simulink model "et_robocon_dev_guy"  (R2013b)
settings: Solver=FixedStepDiscrete  SolverMode=SingleTasking  StartTime=0.0  StopTime=inf  FixedStep=balancer_ts  RelTol=1e-3
undefined symbols (not defined in the file): a_d, a_r, balancerStates_Bus0, Batt, battery_gain, battery_offset, cmd_max, current_mode_status, current_task_operation_status, DiscIntNeverNeededParam, exec_period, Init_Bus0, k_f, k_i, k_phidot, k_thetadot, lightCalib, R, STATE, TRACK_MODE_LIST, ts2, W
libraries: simulink x29, legonxtlib x28, simulink_extras x4, light_sensor_calibration_algorithm_atomic_sub_chart_library x3, gyro_calibration_algorithm_atomic_sub_chart_library x1, limbo_algorithm_atomic_sub_chart_library x1, see_saw x1
(part 3 of 3)

== system et_robocon_dev_guy/Main Controller/normal_operation_modes.line_tracking_mode/line_tracking_mode.processLight/LineTracePID/SwitchController/BasicStage/6thCorner/SpeedUp ==
  TargetFwd : Inport
  LastFwd : Inport  Port=2
  Constant1 : Constant  Value=2  OutDataTypeStr=single  SampleTime=-1
  Saturation1 : Saturate  UpperLimit=160  LowerLimit=80  RndMeth=Simplest
  Sum1 : Sum  Inputs=-+  AccumDataTypeStr=single  OutDataTypeStr=single  RndMeth=Simplest
  Sum2 : Sum  Inputs=|++  AccumDataTypeStr=single  OutDataTypeStr=single  RndMeth=Simplest  InputSameDT=on
  Sum3 : Sum  Inputs=|++  AccumDataTypeStr=single  OutDataTypeStr=single  RndMeth=Simplest  InputSameDT=on
  Switch : Switch  Criteria=u2 > Threshold  OutDataTypeStr=single  RndMeth=Simplest
  Unit Delay1 : UnitDelay  SampleTime=-1
  fwd : Outport
  wires:
  TargetFwd/1 -> Switch/1, Sum1/1
  Switch/1 -> fwd/1
  Sum1/1 -> Switch/2
  Unit Delay1/1 -> Sum2/2
  LastFwd/1 -> Sum3/1
  Constant1/1 -> Sum2/1
  Sum3/1 -> Saturation1/1
  Saturation1/1 -> Switch/3, Sum1/2
  Sum2/1 -> Sum3/2, Unit Delay1/1

== system et_robocon_dev_guy/Main Controller/normal_operation_modes.line_tracking_mode/line_tracking_mode.processLight/LineTracePID/SwitchController/BasicStage/CenterStraight/Normal ==
  note: Max_chargingFwd
  note: speed up (or) speed down counter
  Fwd : Inport
  Constant2 : Constant  Value=0  OutDataTypeStr=single  SampleTime=-1
  Constant4 : Constant  Value=140  OutDataTypeStr=single  SampleTime=-1
  MinMax : MinMax  Function=max
  MinMax1 : MinMax
  Mux : Mux  Inputs=2
  Product : Product  Inputs=*/
  Saturation : Saturate  UpperLimit=10  LowerLimit=-10
  Saturation Dynamic : simulink/Discontinuities/Saturation Dynamic  OutMin=[]  OutMax=[]  OutDataTypeStr=Inherit: Same as second input  OutDataType=fixdt(1, 16)  OutScaling=2^-10  DoSatur=off
  Signal Conversion : SignalConversion
  Sum4 : Sum  Inputs=|+-  AccumDataTypeStr=single  OutDataTypeStr=single  RndMeth=Simplest  InputSameDT=on
  Sum5 : Sum  Inputs=|++  AccumDataTypeStr=single  OutDataTypeStr=single  RndMeth=Simplest  InputSameDT=on
  Unit Delay External IC : simulink/Additional Math & Discrete/Additional Discrete/Unit Delay External IC  tsamp=-1
  steps for rising/falling : Constant  Value=70  OutDataTypeStr=single
  Out1 : Outport
  fwd : Outport  Port=2
  wires:
  Constant2/1 -> Out1/1
  Fwd/1 -> Unit Delay External IC/2, Sum4/2, Mux/2
  Sum4/1 -> Product/1
  Constant4/1 -> Sum4/1, Mux/1
  Sum5/1 -> Saturation Dynamic/2, Unit Delay External IC/1
  Unit Delay External IC/1 -> Sum5/1
  Product/1 -> Saturation/1
  steps for rising/falling/1 -> Product/2
  Mux/1 -> MinMax1/1, MinMax/1
  MinMax/1 -> Saturation Dynamic/1
  MinMax1/1 -> Saturation Dynamic/3
  Saturation/1 -> Sum5/2
  Saturation Dynamic/1 -> Signal Conversion/1
  Signal Conversion/1 -> fwd/1

== system et_robocon_dev_guy/Main Controller/normal_operation_modes.line_tracking_mode/line_tracking_mode.processLight/LineTracePID/SwitchController/BasicStage/CenterStraight/Speak ==
  Enable : EnablePort
  Constant : Constant  Value=50
  Speaker : legonxtlib/Speaker  sinputMode=Volume only  sspeakerFreq=800  sspeakerVolume=50  sspeakerDuration=100
  wires:
  Constant/1 -> Speaker/1

== system et_robocon_dev_guy/Main Controller/normal_operation_modes.line_tracking_mode/line_tracking_mode.processLight/LineTracePID/SwitchController/BasicStage/LastStraight/Normal ==
  note: Max_chargingFwd
  note: speed up (or) speed down counter
  Fwd : Inport
  Constant2 : Constant  Value=0  OutDataTypeStr=single  SampleTime=-1
  Constant4 : Constant  Value=140  OutDataTypeStr=single  SampleTime=-1
  MinMax : MinMax  Function=max
  MinMax1 : MinMax
  Mux : Mux  Inputs=2
  Product : Product  Inputs=*/
  Saturation : Saturate  UpperLimit=10  LowerLimit=-10
  Saturation Dynamic : simulink/Discontinuities/Saturation Dynamic  OutMin=[]  OutMax=[]  OutDataTypeStr=Inherit: Same as second input  OutDataType=fixdt(1, 16)  OutScaling=2^-10  DoSatur=off
  Signal Conversion : SignalConversion
  Sum4 : Sum  Inputs=|+-  AccumDataTypeStr=single  OutDataTypeStr=single  RndMeth=Simplest  InputSameDT=on
  Sum5 : Sum  Inputs=|++  AccumDataTypeStr=single  OutDataTypeStr=single  RndMeth=Simplest  InputSameDT=on
  Unit Delay External IC : simulink/Additional Math & Discrete/Additional Discrete/Unit Delay External IC  tsamp=-1
  steps for rising/falling : Constant  Value=60  OutDataTypeStr=single
  Out1 : Outport
  fwd : Outport  Port=2
  wires:
  Constant2/1 -> Out1/1
  Fwd/1 -> Unit Delay External IC/2, Sum4/2, Mux/2
  Sum4/1 -> Product/1
  Constant4/1 -> Sum4/1, Mux/1
  Sum5/1 -> Saturation Dynamic/2, Unit Delay External IC/1
  Unit Delay External IC/1 -> Sum5/1
  Product/1 -> Saturation/1
  steps for rising/falling/1 -> Product/2
  Mux/1 -> MinMax1/1, MinMax/1
  MinMax/1 -> Saturation Dynamic/1
  MinMax1/1 -> Saturation Dynamic/3
  Saturation/1 -> Sum5/2
  Saturation Dynamic/1 -> Signal Conversion/1
  Signal Conversion/1 -> fwd/1

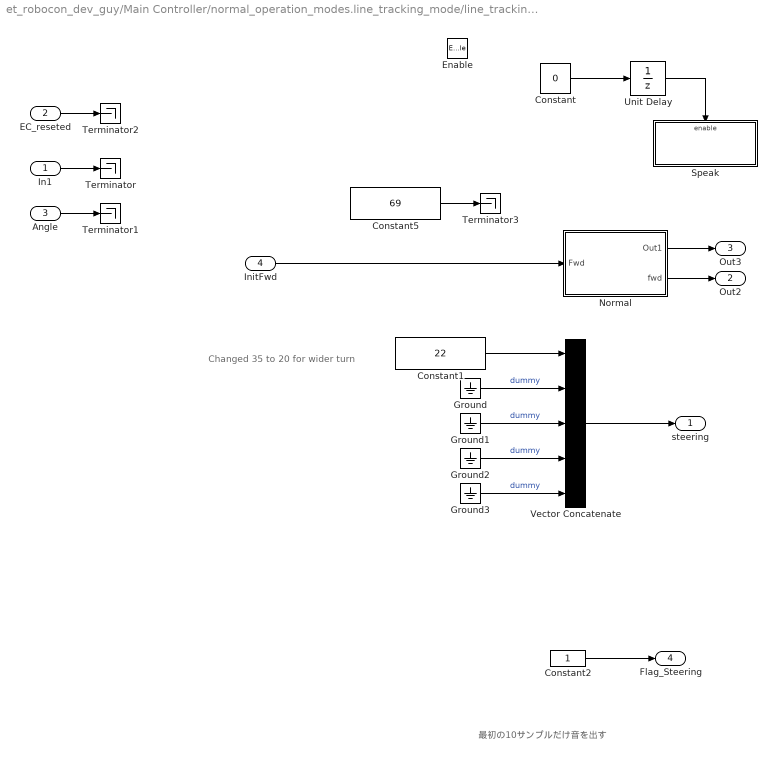
== system et_robocon_dev_guy/Main Controller/normal_operation_modes.line_tracking_mode/line_tracking_mode.processLight/LineTracePID/SwitchController/BasicStage/ShortCut/BlindRun ==
  note: Changed 35 to 20 for wider turn
  note: 最初の10サンプルだけ音を出す
  In1 : Inport
  EC_reseted : Inport  Port=2
  Angle : Inport  Port=3
  InitFwd : Inport  Port=4
  Enable : EnablePort
  Constant : Constant  Value=0
  Constant1 : Constant  Value=22  OutDataTypeStr=single  SampleTime=-1
  Constant2 : Constant  OutDataTypeStr=single  SampleTime=-1
  Constant5 : Constant  Value=69  OutDataTypeStr=single  SampleTime=-1
  Ground{,1..3} (4 alike) : Ground
  Normal : Subsystem  TreatAsAtomicUnit=on
  Speak : Subsystem  TreatAsAtomicUnit=on
  Terminator{,1..3} (4 alike) : Terminator
  Unit Delay : UnitDelay  InitialCondition=1  SampleTime=-1
  Vector Concatenate : Concatenate  NumInputs=5
  steering : Outport
  Out2 : Outport  Port=2
  Out3 : Outport  Port=3
  Flag_Steering : Outport  Port=4
  wires:
  In1/1 -> Terminator/1
  Angle/1 -> Terminator1/1
  EC_reseted/1 -> Terminator2/1
  Normal/2(fwd) -> Out2/1
  Normal/1(Out1) -> Out3/1
  Vector Concatenate/1 -> steering/1
  Ground/1 -> Vector Concatenate/2  "dummy"
  Ground1/1 -> Vector Concatenate/3  "dummy"
  Ground2/1 -> Vector Concatenate/4  "dummy"
  Ground3/1 -> Vector Concatenate/5  "dummy"
  Constant2/1 -> Flag_Steering/1
  Constant5/1 -> Terminator3/1
  InitFwd/1 -> Normal/1(Fwd)
  Constant1/1 -> Vector Concatenate/1
  Constant/1 -> Unit Delay/1
  Unit Delay/1 -> Speak/Enable

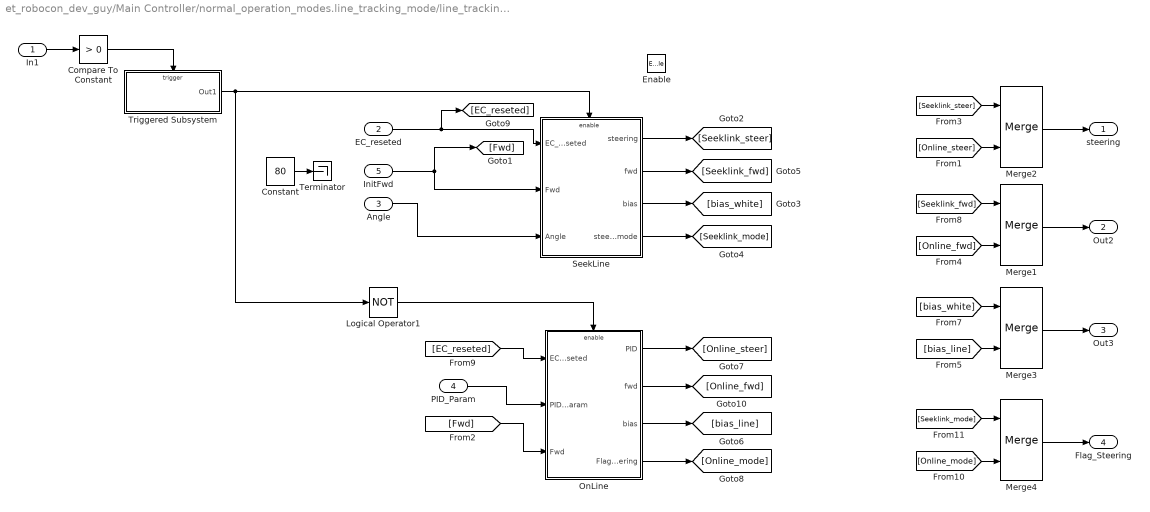
== system et_robocon_dev_guy/Main Controller/normal_operation_modes.line_tracking_mode/line_tracking_mode.processLight/LineTracePID/SwitchController/BasicStage/ShortCut/SeekAndPIDRun ==
  In1 : Inport
  EC_reseted : Inport  Port=2
  Angle : Inport  Port=3
  PID_Param : Inport  Port=4
  InitFwd : Inport  Port=5
  Enable : EnablePort
  Compare To Constant : simulink/Logic and Bit Operations/Compare To Constant  relop=>  const=0  OutDataTypeStr=boolean
  Constant : Constant  Value=80  OutDataTypeStr=single
  Logical Operator1 : Logic  Operator=NOT  AllPortsSameDT=off  OutDataTypeStr=boolean
  Merge{1..4} (4 alike) : Merge
  OnLine : Subsystem  TreatAsAtomicUnit=on
  SeekLine : Subsystem  TreatAsAtomicUnit=on
  Terminator : Terminator
  Triggered Subsystem : Subsystem  TreatAsAtomicUnit=on
  steering : Outport
  Out2 : Outport  Port=2
  Out3 : Outport  Port=3
  Flag_Steering : Outport  Port=4
  wires:
  [bias_line] -> Merge3/2
  [bias_white] -> Merge3/1
  OnLine/3(bias) -> [bias_line]
  SeekLine/3(bias) -> [bias_white]
  PID_Param/1 -> OnLine/2(PID_Param)
  [EC_reseted] -> OnLine/1(EC_reseted)
  Logical Operator1/1 -> OnLine/Enable
  Angle/1 -> SeekLine/3(Angle)
  EC_reseted/1 -> SeekLine/1(EC_reseted), [EC_reseted]
  Merge1/1 -> Out2/1
  Merge3/1 -> Out3/1
  Merge2/1 -> steering/1
  Merge4/1 -> Flag_Steering/1
  Compare To Constant/1 -> Triggered Subsystem/Trigger
  Triggered Subsystem/1(Out1) -> SeekLine/Enable, Logical Operator1/1
  [Fwd] -> OnLine/3(Fwd)
  In1/1 -> Compare To Constant/1
  SeekLine/1(steering) -> [Seeklink_steer]
  SeekLine/2(fwd) -> [Seeklink_fwd]
  SeekLine/4(steering_mode) -> [Seeklink_mode]
  [Seeklink_steer] -> Merge2/1
  [Online_steer] -> Merge2/2
  [Seeklink_fwd] -> Merge1/1
  [Online_fwd] -> Merge1/2
  [Seeklink_mode] -> Merge4/1
  [Online_mode] -> Merge4/2
  OnLine/1(PID) -> [Online_steer]
  OnLine/2(fwd) -> [Online_fwd]
  OnLine/4(Flag_Steering) -> [Online_mode]
  InitFwd/1 -> [Fwd], SeekLine/2(Fwd)
  Constant/1 -> Terminator/1

== system et_robocon_dev_guy/Main Controller/normal_operation_modes.line_tracking_mode/line_tracking_mode.processLight/LineTracePID/SwitchController/BasicStage/ShortCut/Triggered Subsystem ==
  Trigger : TriggerPort
  Constant : Constant  Value=0  OutDataTypeStr=boolean
  Out1 : Outport  InitialOutput=[1]
  wires:
  Constant/1 -> Out1/1

== system et_robocon_dev_guy/Main Controller/normal_operation_modes.line_tracking_mode/line_tracking_mode.processLight/LineTracePID/SwitchController/BasicStage/Slope/Slope Mode 0 ==
  Fwd : Inport
  Bias : Inport  Port=2
  Action Port : ActionPort  ActionType=default
  bias : Outport
  fwd : Outport  Port=2
  wires:
  Bias/1 -> bias/1
  Fwd/1 -> fwd/1

== system et_robocon_dev_guy/Main Controller/normal_operation_modes.line_tracking_mode/line_tracking_mode.processLight/LineTracePID/SwitchController/BasicStage/Slope/Slope Mode 1 ==
  Fwd : Inport
  Bias : Inport  Port=2
  PreFwd : Inport  Port=3
  Action Port : ActionPort  ActionType=case
  Constant : Constant  Value=-1  OutDataTypeStr=single
  Saturation Dynamic : simulink/Discontinuities/Saturation Dynamic  OutMin=[]  OutMax=[]  OutDataTypeStr=Inherit: Same as second input  OutDataType=fixdt(1, 16)  OutScaling=2^-10  DoSatur=off
  Signal Conversion : SignalConversion
  Sum : Sum  Inputs=|++
  Sum1 : Sum  Inputs=|++
  Unit Delay : UnitDelay  SampleTime=-1
  bias : Outport
  fwd : Outport  Port=2
  wires:
  Bias/1 -> bias/1
  Fwd/1 -> Saturation Dynamic/3
  Constant/1 -> Sum/1
  Sum/1 -> Unit Delay/1, Sum1/2
  Sum1/1 -> Saturation Dynamic/2
  Saturation Dynamic/1 -> Signal Conversion/1
  PreFwd/1 -> Saturation Dynamic/1, Sum1/1
  Signal Conversion/1 -> fwd/1
  Unit Delay/1 -> Sum/2

== system et_robocon_dev_guy/Main Controller/normal_operation_modes.line_tracking_mode/line_tracking_mode.processLight/LineTracePID/SwitchController/BasicStage/Slope/Slope Mode 2 ==
  Fwd : Inport
  Bias : Inport  Port=2
  PreFwd : Inport  Port=3
  Action Port : ActionPort  ActionType=case
  Constant : Constant  OutDataTypeStr=single
  Saturation Dynamic : simulink/Discontinuities/Saturation Dynamic  OutMin=[]  OutMax=[]  OutDataTypeStr=Inherit: Same as second input  OutDataType=fixdt(1, 16)  OutScaling=2^-10  DoSatur=off
  Signal Conversion : SignalConversion
  Sum : Sum  Inputs=|++
  Sum1 : Sum  Inputs=|++
  Unit Delay : UnitDelay  SampleTime=-1
  bias : Outport
  fwd : Outport  Port=2
  wires:
  Bias/1 -> bias/1
  Constant/1 -> Sum/1
  Sum/1 -> Unit Delay/1, Sum1/2
  Sum1/1 -> Saturation Dynamic/2
  Saturation Dynamic/1 -> Signal Conversion/1
  PreFwd/1 -> Saturation Dynamic/1, Sum1/1
  Fwd/1 -> Saturation Dynamic/3
  Signal Conversion/1 -> fwd/1
  Unit Delay/1 -> Sum/2

== system et_robocon_dev_guy/Main Controller/normal_operation_modes.line_tracking_mode/line_tracking_mode.processLight/LineTracePID/SwitchController/BonusStage/Gate/Normal ==
  Fwd : Inport
  Constant2 : Constant  Value=-10  OutDataTypeStr=single  SampleTime=-1
  Out1 : Outport
  fwd : Outport  Port=2
  wires:
  Fwd/1 -> fwd/1
  Constant2/1 -> Out1/1

== system et_robocon_dev_guy/Main Controller/normal_operation_modes.line_tracking_mode/line_tracking_mode.processLight/LineTracePID/SwitchController/BonusStage/Gate/SlowDown ==
  TargetFwd : Inport
  LastFwd : Inport  Port=2
  Constant1 : Constant  Value=-0.5  OutDataTypeStr=single  SampleTime=-1
  Saturation1 : Saturate  UpperLimit=160  LowerLimit=0  RndMeth=Simplest
  Sum1 : Sum  Inputs=+-  AccumDataTypeStr=single  OutDataTypeStr=single  RndMeth=Simplest
  Sum2 : Sum  Inputs=|++  AccumDataTypeStr=single  OutDataTypeStr=single  RndMeth=Simplest  InputSameDT=on
  Sum3 : Sum  Inputs=|++  AccumDataTypeStr=single  OutDataTypeStr=single  RndMeth=Simplest  InputSameDT=on
  Switch : Switch  Criteria=u2 > Threshold  OutDataTypeStr=single  RndMeth=Simplest
  Unit Delay1 : UnitDelay  SampleTime=-1
  fwd : Outport
  wires:
  TargetFwd/1 -> Switch/1, Sum1/1
  Switch/1 -> fwd/1
  Sum1/1 -> Switch/2
  Unit Delay1/1 -> Sum2/2
  LastFwd/1 -> Sum3/1
  Constant1/1 -> Sum2/1
  Sum3/1 -> Saturation1/1
  Saturation1/1 -> Switch/3, Sum1/2
  Sum2/1 -> Sum3/2, Unit Delay1/1

== system et_robocon_dev_guy/Main Controller/normal_operation_modes.line_tracking_mode/line_tracking_mode.processLight/LineTracePID/SwitchController/BonusStage/IntoGarage/Normal ==
  Fwd : Inport
  Constant2 : Constant  Value=-10  OutDataTypeStr=single  SampleTime=-1
  Out1 : Outport
  fwd : Outport  Port=2
  wires:
  Constant2/1 -> Out1/1
  Fwd/1 -> fwd/1

== system et_robocon_dev_guy/Main Controller/normal_operation_modes.line_tracking_mode/line_tracking_mode.processLight/LineTracePID/SwitchController/BasicStage/ShortCut/BlindRun/Normal ==
  Fwd : Inport
  Constant2 : Constant  Value=0  OutDataTypeStr=single  SampleTime=-1
  Out1 : Outport
  fwd : Outport  Port=2
  wires:
  Constant2/1 -> Out1/1
  Fwd/1 -> fwd/1

== system et_robocon_dev_guy/Main Controller/normal_operation_modes.line_tracking_mode/line_tracking_mode.processLight/LineTracePID/SwitchController/BasicStage/ShortCut/BlindRun/Speak ==
  Enable : EnablePort
  Constant : Constant  Value=50
  Speaker : legonxtlib/Speaker  sinputMode=Volume only  sspeakerFreq=800  sspeakerVolume=50  sspeakerDuration=100
  wires:
  Constant/1 -> Speaker/1

== system et_robocon_dev_guy/Main Controller/normal_operation_modes.line_tracking_mode/line_tracking_mode.processLight/LineTracePID/SwitchController/BasicStage/ShortCut/SeekAndPIDRun/OnLine ==
  note: 最初の10サンプルだけ音を出す
  EC_reseted : Inport
  PID_Param : Inport  Port=2
  Fwd : Inport  Port=3
  Enable : EnablePort
  Constant : Constant  Value=0.2  OutDataTypeStr=single
  Constant1 : Constant  Value=0  OutDataTypeStr=single  SampleTime=-1
  Constant2 : Constant  Value=5  OutDataTypeStr=single  SampleTime=-1
  Constant3 : Constant  Value=0
  Saturation : Saturate  UpperLimit=140  LowerLimit=0
  Speak : Subsystem  TreatAsAtomicUnit=on
  Sum : Sum  Inputs=|++
  Sum1 : Sum  Inputs=|++
  Terminator : Terminator
  Unit Delay : UnitDelay  SampleTime=-1
  Unit Delay1 : UnitDelay  InitialCondition=1  SampleTime=-1
  PID : Outport
  fwd : Outport  Port=2
  bias : Outport  Port=3
  Flag_Steering : Outport  Port=4
  wires:
  Constant2/1 -> bias/1
  PID_Param/1 -> PID/1
  EC_reseted/1 -> Terminator/1
  Fwd/1 -> Sum1/1
  Sum1/1 -> Saturation/1
  Sum/1 -> Unit Delay/1, Sum1/2
  Unit Delay/1 -> Sum/2
  Saturation/1 -> fwd/1
  Constant1/1 -> Flag_Steering/1
  Constant/1 -> Sum/1
  Constant3/1 -> Unit Delay1/1
  Unit Delay1/1 -> Speak/Enable

== system et_robocon_dev_guy/Main Controller/normal_operation_modes.line_tracking_mode/line_tracking_mode.processLight/LineTracePID/SwitchController/BasicStage/ShortCut/SeekAndPIDRun/SeekLine ==
  note: Change -7 to -3
  EC_reseted : Inport
  Fwd : Inport  Port=2
  Angle : Inport  Port=3
  Enable : EnablePort
  Constant : Constant  Value=-3  OutDataTypeStr=single
  Constant1 : Constant  OutDataTypeStr=single  SampleTime=-1
  Constant2 : Constant  Value=0  OutDataTypeStr=single  SampleTime=-1
  Constant3 : Constant  Value=-10  OutDataTypeStr=single
  Constant4 : Constant  Value=0
  Ground{,1..3} (4 alike) : Ground
  Speak : Subsystem  TreatAsAtomicUnit=on
  Terminator : Terminator
  Terminator1 : Terminator
  Terminator2 : Terminator
  Unit Delay : UnitDelay  InitialCondition=1  SampleTime=-1
  Vector Concatenate : Concatenate  NumInputs=5
  steering : Outport
  fwd : Outport  Port=2
  bias : Outport  Port=3
  steering_mode : Outport  Port=4
  wires:
  Angle/1 -> Terminator1/1
  EC_reseted/1 -> Terminator/1
  Fwd/1 -> fwd/1
  Constant2/1 -> bias/1
  Ground/1 -> Vector Concatenate/2  "dummy"
  Ground1/1 -> Vector Concatenate/3  "dummy"
  Ground2/1 -> Vector Concatenate/4  "dummy"
  Ground3/1 -> Vector Concatenate/5  "dummy"
  Vector Concatenate/1 -> steering/1
  Constant1/1 -> steering_mode/1
  Constant/1 -> Vector Concatenate/1
  Constant3/1 -> Terminator2/1
  Constant4/1 -> Unit Delay/1
  Unit Delay/1 -> Speak/Enable

== system et_robocon_dev_guy/Main Controller/normal_operation_modes.line_tracking_mode/line_tracking_mode.processLight/LineTracePID/SwitchController/BasicStage/ShortCut/SeekAndPIDRun/Triggered Subsystem ==
  Trigger : TriggerPort
  Constant : Constant  Value=0  OutDataTypeStr=boolean
  Out1 : Outport  InitialOutput=[1]
  wires:
  Constant/1 -> Out1/1

== system et_robocon_dev_guy/Main Controller/normal_operation_modes.line_tracking_mode/line_tracking_mode.processLight/LineTracePID/SwitchController/BasicStage/ShortCut/SeekAndPIDRun/OnLine/Speak ==
  Enable : EnablePort
  Constant : Constant  Value=50
  Speaker : legonxtlib/Speaker  sinputMode=Volume only  sspeakerFreq=800  sspeakerVolume=50  sspeakerDuration=100
  wires:
  Constant/1 -> Speaker/1

== system et_robocon_dev_guy/Main Controller/normal_operation_modes.line_tracking_mode/line_tracking_mode.processLight/LineTracePID/SwitchController/BasicStage/ShortCut/SeekAndPIDRun/SeekLine/Speak ==
  Enable : EnablePort
  Constant : Constant  Value=50
  Speaker : legonxtlib/Speaker  sinputMode=Volume only  sspeakerFreq=800  sspeakerVolume=50  sspeakerDuration=100
  wires:
  Constant/1 -> Speaker/1

== stateflow chart et_robocon_dev_guy/State Estimation/Gyro Processing/Reset Subsystem ==
  state CheckForReset
    bind: doProcess;
    entry: doProcess;
    during: doProcess;
  (default) -> CheckForReset
  CheckForReset -> CheckForReset : [init_flag == 1]
  data: init_flag input
  events: doProcess output FUNCTION_CALL_EVENT

== stateflow chart et_robocon_dev_guy/Main Controller/normal_operation_modes.line_tracking_mode ==
  state line_tracking_mode
    entry:
    desired_tail = single(0); %radian
    entry, during:
    PWM.tail = tail_controller(sensors.theta_T,desired_tail);
    exit:
    PWM.tail = single(0);
    state Waiting
      entry: debugFlag = uint16(400);
    state Track
      entry:
      debugFlag = uint16(401);
      during:
      on every(3, tick):  lineTrackCmd = processLight(rawSensors);
      during:
      [PWM.left PWM.right] = balanceControl(rawSensors,lineTrackCmd);
    state Stop
      entry:
      speed_ref = lineTrackCmd(1);
      during:
      lineTrackCmd = single([speed_ref 0]');
      [PWM.left PWM.right] = balanceControl(rawSensors,lineTrackCmd);
      desired_tail = single(1.6); %radian
      speed_ref = speed_ref - single(1);
    state Kick
      entry:
      PWM.left = single(100)
      PWM.right = single(100);
      exit:
      PWM.left = single(0)
      PWM.right = single(0);
    state Done
      entry:
      turnLightOn;
      debugFlag = uint16(402);
      PWM.left = single(0); PWM.right = single(0);
      current_mode_status = OperationModeStatusEnum.SUCCESSFULLY_COMPLETED;
    state turnLightOn [function]
    state lineTrackCmd = processLight(rawSensors) [function]
    state [leftPWM,rightPWM]  = balanceControl(rawSensors, lineTrackCmd) [function]
    state cmd = tail_controller(current,desired) [function]
    (default) -> Waiting
    Waiting -> Track : [hasChangedFrom(touch,single(0))]
    Track -> Stop : [(sensors.theta_L + sensors.theta_R)/2>single(320)]
    Stop -> Kick : [speed_ref<0]
    Kick -> Done : after(0.2,sec)
  data: lineTrackCmd function_output single size=2; rawSensors function_input Bus: Sensors_Bus size=1; leftPWM function_output single size=1; rawSensors function_input Bus: Sensors_Bus size=1; rightPWM function_output; lineTrackCmd function_input single size=2; current function_input single size=1; desired function_input single size=1; cmd function_output single size=1; sensors input Bus: Sensors_Bus size=1; lightCalib data_store_memory size=1; touch input single size=1; PWM output Bus: PWM_bus size=1; debugFlag output uint16 size=1; current_mode_status data_store_memory; desired_tail local single size=1; speed_ref local single size=1; states input Bus: States_Bus size=1; rawSensors input Bus: Sensors_Bus size=1; lineTrackCmd local single size=2

== stateflow chart et_robocon_dev_guy/State Estimation/StateEstimation/Reset Subsystem ==
  state CheckForReset
    bind: doProcess;
    entry: doProcess;
    during: doProcess;
  (default) -> CheckForReset
  CheckForReset -> CheckForReset : [init_flag == 1]
  data: init_flag input
  events: doProcess output FUNCTION_CALL_EVENT

== stateflow chart et_robocon_dev_guy/Main Controller ==
  state restore
  state emergency_stop
    entry:
    debugFlag = uint16(9999);
  state normal_operation_modes
    state gyro_calibration_mode
    state light_calibration_on_tail
    state light_calibration_up
    state line_tracking_mode
    state see_saw
    state limbo_mode
    state light_calibration_limbo
    state WeShouldNotBeHere
    (default) -> (junction 12) : {
        | current_mode_status = OperationModeStatusEnum.IN_PROGRESS;
        | }
    (junction 12) -> gyro_calibration_mode [order 1] : [  current_mode == OperationModeEnum.GYRO_CALIBRATION ]
    (junction 12) -> (junction 13) [order 2]
    (junction 13) -> light_calibration_on_tail [order 1] : [ current_mode == OperationModeEnum.LIGHT_CALIBRATION_ON_TAIL ]
    (junction 13) -> (junction 144) [order 2]
    (junction 144) -> light_calibration_up [order 1] : [ current_mode == OperationModeEnum.LIGHT_CALIBRATION_UP ]
    (junction 144) -> (junction 14) [order 2]
    (junction 14) -> line_tracking_mode [order 1] : [ current_mode == OperationModeEnum.LINE_TRACKING ]
    (junction 14) -> (junction 15) [order 2]
    (junction 15) -> see_saw [order 1] : [ current_mode == OperationModeEnum.SEE_SAW ]
    (junction 15) -> (junction 17) [order 2]
    (junction 17) -> limbo_mode [order 1] : [  current_mode == OperationModeEnum.LIMBO ]
    (junction 17) -> (junction 19) [order 2]
    (junction 19) -> light_calibration_limbo [order 1] : [ current_mode == OperationModeEnum.LIGHT_CALIBRATION_LIMBO ]
    (junction 19) -> (junction 140) [order 2]
    (junction 140) -> ? [order 1] : [ current_mode == OperationModeEnum.SEE_SAW_PRINCESS ]
    (junction 140) -> (junction 154) [order 1]
    (junction 154) -> ? [order 1] : [ current_mode == OperationModeEnum.YOSHI ]
    (junction 154) -> (junction 99) [order 1]
    (junction 99) -> WeShouldNotBeHere
  (default) -> (junction 38) : {initFlags = Init_Bus0;BT_status_out = single(0)}
  (junction 37) -> (junction 38)
  (junction 43) -> (junction 37)
  (junction 38) -> (junction 39) : { current_mode_index = uint8( 0 ); }
  (junction 40) -> (junction 39)
  restore -> (junction 40) : [ false == touch ]
  (junction 39) -> (junction 41) : {
      | current_mode_status = OperationModeStatusEnum.NOT_STARTED;
      | }
  normal_operation_modes -> (junction 40) [order 2] : [ current_mode_status == OperationModeStatusEnum.SUCCESSFULLY_COMPLETED ]
  (junction 42) -> (junction 41)
  (junction 41) -> (junction 44) : { current_mode_index = current_mode_index + uint8( 1 ); }
  (junction 47) -> (junction 42)
  emergency_stop -> restore : [ true == touch ]
  (junction 44) -> (junction 43) [order 1] : [ numel( TRACK_MODE_LIST ) < current_mode_index ]
      | % If the "current_mode_index" has exceeded the number
      | % of elements in the list, it should "wrap" back to the start.
  (junction 44) -> (junction 45) [order 2]
  (junction 45) -> (junction 46) : {
      | current_mode = TRACK_MODE_LIST( current_mode_index );
      | }
  (junction 46) -> (junction 47) [order 1] : [  current_mode == OperationModeEnum.SKIP ]
  (junction 46) -> normal_operation_modes [order 2]
  normal_operation_modes -> emergency_stop [order 1] : [ true == fall_detection_input ]
      | {current_mode_status = OperationModeStatusEnum.ABORTED;}
  data: rawSensors input Bus: Sensors_Bus size=1; PWM output Bus: PWM_bus size=1; TRACK_MODE_LIST parameter Enum: OperationModeEnum; current_mode_index local uint8; current_mode data_store_memory; states input Bus: States_Bus size=1; fall_detection_input input boolean size=1; current_mode_status data_store_memory; sensors input Bus: Sensors_Bus size=1; lightCalib data_store_memory; debugFlag output uint16 size=1; BT_status_out output single size=1; touch input single size=1; initFlags output Bus: Init_Bus size=1; Init_Bus0 parameter Bus: Init_Bus size=1; balancerStates_Bus0 parameter Bus: Balancer_States_Bus size=1
